simulink model "optimalswitching"  (R2024b)
settings: Solver=ode45  StartTime=0.0  StopTime=0.5  MaxStep=1e-7  MinStep=1e-8  RelTol=1e-6
values from neighbouring files (symbols this model uses):
  ma = 0.1    [three_level_parameter.m]
  Ts = 1/Fsw    (= 0.00111111111111)    [three_level_parameter.m]
  Vd = 400    [three_level_parameter.m]
  Vrefmax = Vdclink_max*cos(pi/6)    [three_level_parameter.m]
libraries: spsIGBTDiodeLib x12, spsDiodeLib x6, spsSeriesRLCLoadLib x3, spsDCVoltageSourceLib x2, spsGroundLib x1, spsThreePhaseVIMeasurementLib x1, sps_lib x1, simulink x1
settings SolverCC: ZeroCrossControl=DisableAll
settings DataIOCC: Refine=1000

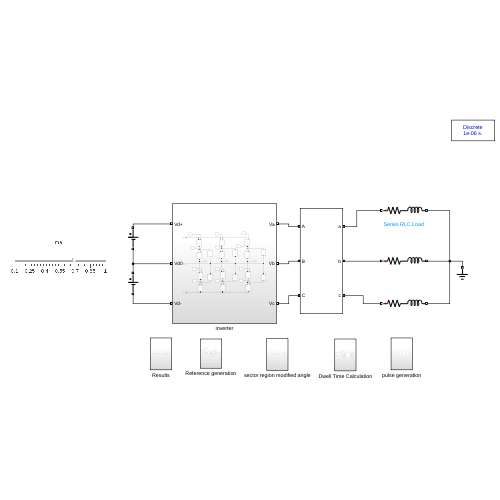
[thumbnail: Simulink's stored preview of the top-level diagram]
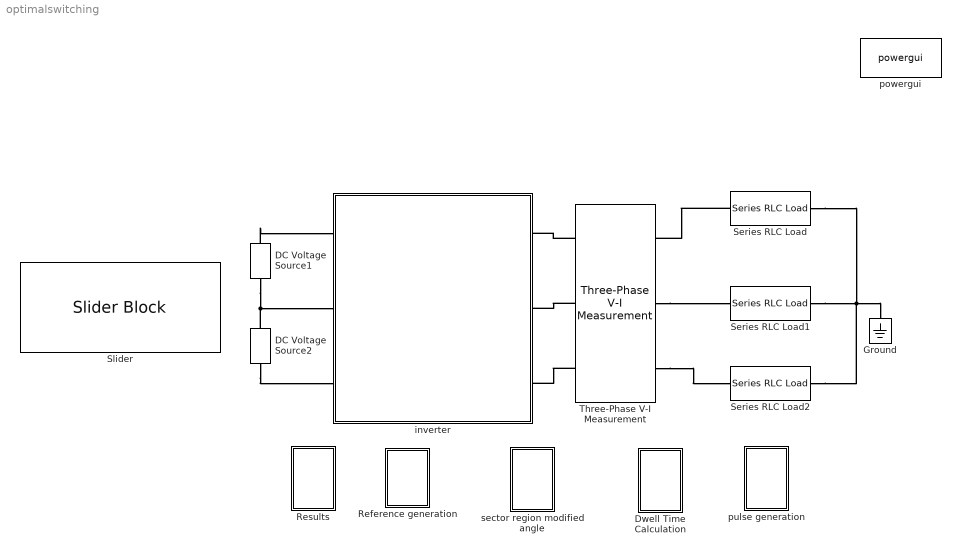
== system optimalswitching ==
  DC Voltage Source1 : spsDCVoltageSourceLib/DC Voltage Source  Amplitude=200  Measurements=None
  DC Voltage Source2 : spsDCVoltageSourceLib/DC Voltage Source  Amplitude=200  Measurements=None
  Dwell Time Calculation : Subsystem
  Ground : spsGroundLib/Ground  LConnTagsString=a
  Reference generation : Subsystem
  Results : Subsystem
  Series RLC Load : spsSeriesRLCLoadLib/Series RLC Load  LConnTagsString=a  RConnTagsString=__new0  NominalVoltage=240  NominalFrequency=50  ActivePower=1e3  InductivePower=484  CapacitivePower=0  Setx0=off  InitialVoltage=0  SetiL0=off  InitialCurrent=0  Measurements=None  LoadType=constant Z
  Series RLC Load1 : spsSeriesRLCLoadLib/Series RLC Load  LConnTagsString=a  RConnTagsString=__new0  NominalVoltage=240  NominalFrequency=50  ActivePower=1e3  InductivePower=484  CapacitivePower=0  Setx0=off  InitialVoltage=0  SetiL0=off  InitialCurrent=0  Measurements=None  LoadType=constant Z
  Series RLC Load2 : spsSeriesRLCLoadLib/Series RLC Load  LConnTagsString=a  RConnTagsString=__new0  NominalVoltage=240  NominalFrequency=50  ActivePower=1e3  InductivePower=484  CapacitivePower=0  Setx0=off  InitialVoltage=0  SetiL0=off  InitialCurrent=0  Measurements=None  LoadType=constant Z
  Slider : SliderBlock  ScaleMin=0.1  ScaleMax=1
  Three-Phase V-I Measurement : spsThreePhaseVIMeasurementLib/Three-Phase V-I Measurement  VoltageMeasurement=phase-to-ground  SetLabelV=on  LabelV=Vabc  Vpu=off  VpuLL=off  CurrentMeasurement=yes  SetLabelI=on  LabelI=Iabc  Ipu=off  Pbase=100e6  Vbase=500e3  OutputType=Complex  PhasorSimulation=off  PSBequivalent=0
  inverter : Subsystem
  powergui : sps_lib/powergui  Priority=1  SimulationMode=Discrete  SampleTime=1e-6  frequency=60  Iterations=50  frequencyindice=0  Pbase=100e6  ErrMax=1e-4  UnitsV=kV  UnitsW=MW  buscounter=0  FunctionMessages=off  echomessages=off  EnableUseOfTLC=off  CurrentSourceSwitches=off  DisableSnubberDevices=off  DisableRonSwitches=off  DisableVfSwitches=off  DisplayEquations=off  AutomaticDiscreteSolvers=off  SolverType=Tustin/Backward Euler (TBE)  Interpol=off  ExternalGateDelay=off  methode=off  Ts=100  x0status=blocks  SPID=on  SwTol=0  HookPort=off  NonlinearTolerance=1e-4  nMaxIteration=100  ContinueOnMaxIteration=off  RestoreLinks=warning  ResistiveCurrentMeasurement=off  Frange=[0:2:500]  Ylog=off  Xlog=on  ShowGrid=off  save=off  variable=ZData  structure=0  ZoomFFT=off  StartTime=0.0  cycles=1  DisplayStyle=1  fundamental=60  FreqAxis=off  MaxFrequency=1000  frequencyindicesteady=1  RmsSteady=1  display=off
  pulse generation : Subsystem
  sector region modified angle : Subsystem
  connections:
  Series RLC Load1/RConn1 -- Series RLC Load/RConn1 -- Ground/LConn1 -- Series RLC Load2/RConn1
  Three-Phase V-I Measurement/RConn3 -- Series RLC Load2/LConn1
  Series RLC Load/LConn1 -- Three-Phase V-I Measurement/RConn1
  Three-Phase V-I Measurement/RConn2 -- Series RLC Load1/LConn1
  Three-Phase V-I Measurement/LConn1 -- inverter/RConn1
  Three-Phase V-I Measurement/LConn2 -- inverter/RConn2
  Three-Phase V-I Measurement/LConn3 -- inverter/RConn3
  DC Voltage Source1/RConn1 -- inverter/LConn1
  DC Voltage Source1/LConn1 -- DC Voltage Source2/RConn1 -- inverter/LConn2
  DC Voltage Source2/LConn1 -- inverter/LConn3

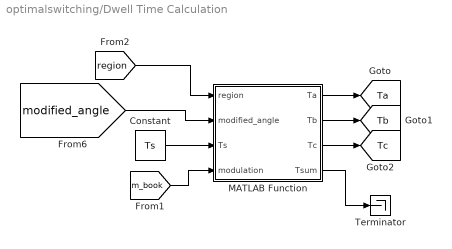
== system optimalswitching/Dwell Time Calculation ==
  Constant : Constant  Value=Ts
  MATLAB Function : MATLAB Function  TreatAsAtomicUnit=on
  Terminator : Terminator
  tag scope: Ta=global, Tb=global, Tc=global
  wires:
  [m_book] -> MATLAB Function/4(modulation)
  [region] -> MATLAB Function/1(region)
  Constant/1 -> MATLAB Function/3(Ts)
  [modified_angle] -> MATLAB Function/2(modified_angle)
  MATLAB Function/1(Ta) -> [Ta]
  MATLAB Function/2(Tb) -> [Tb]
  MATLAB Function/3(Tc) -> [Tc]
  MATLAB Function/4(Tsum) -> Terminator/1

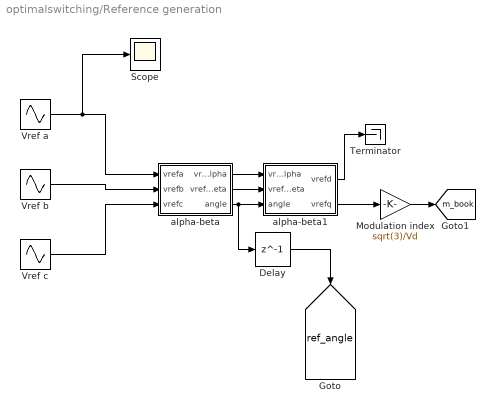
== system optimalswitching/Reference generation ==
  Delay : Delay  DelayLength=1  InitialCondition=0  SampleTime=Ts
  Modulation index : Gain  Gain=sqrt(3)/Vd
  Scope : Scope
  Terminator : Terminator
  Vref a : Sin  Amplitude=ma*Vrefmax  Frequency=2*pi*50  SampleTime=0
  Vref b : Sin  Amplitude=ma*Vrefmax  Frequency=2*pi*50  Phase=4*pi/3  SampleTime=0
  Vref c : Sin  Amplitude=ma*Vrefmax  Frequency=2*pi*50  Phase=2*pi/3  SampleTime=0
  alpha-beta : MATLAB Function  TreatAsAtomicUnit=on
  alpha-beta1 : MATLAB Function  TreatAsAtomicUnit=on
  tag scope: m_book=global, ref_angle=global
  wires:
  alpha-beta1/2(vrefq) -> Modulation index/1
  Vref b/1 -> alpha-beta/2(vrefb)
  alpha-beta/2(vrefbeta) -> alpha-beta1/2(vrefbeta)
  Vref c/1 -> alpha-beta/3(vrefc)
  Vref a/1 -> Scope/1, alpha-beta/1(vrefa)
  alpha-beta/3(angle) -> Delay/1, alpha-beta1/3(angle)
  Modulation index/1 -> [m_book]
  alpha-beta/1(vrefalpha) -> alpha-beta1/1(vrefalpha)
  alpha-beta1/1(vrefd) -> Terminator/1
  Delay/1 -> [ref_angle]

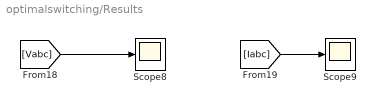
== system optimalswitching/Results ==
  Scope8 : Scope
  Scope9 : Scope
  wires:
  [Iabc] -> Scope9/1
  [Vabc] -> Scope8/1

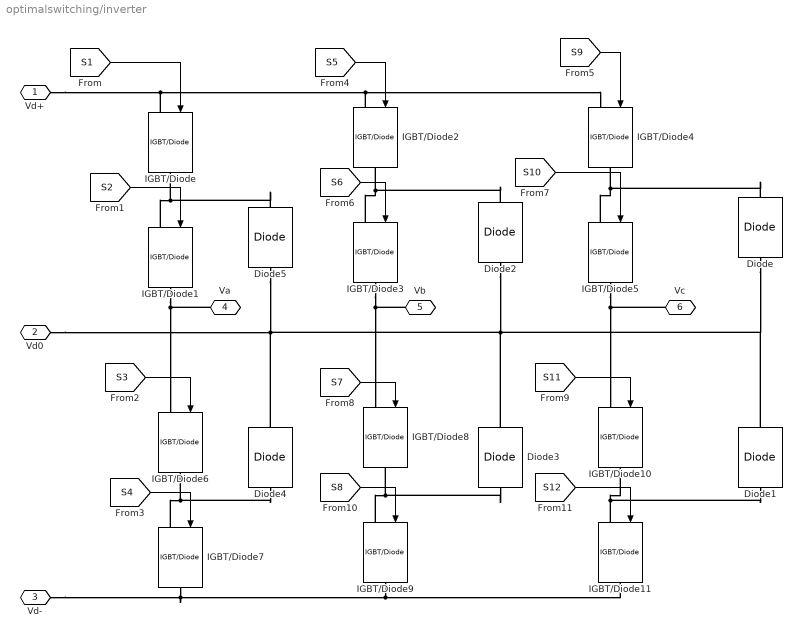
== system optimalswitching/inverter ==
  Diode{,1..5} (6 alike) : spsDiodeLib/Diode  Ron=0.001  Lon=0  Vf=0.8  IC=0  UseSnubber=0  Rs=500  Cs=250e-9  Measurements=off
  IGBT/Diode{,1..11} (12 alike) : spsIGBTDiodeLib/IGBT//Diode  Ron=1e-3  Rs=1e5  Cs=inf  Measurements=off
  Vd+ : PMIOPort  Side=Left
  Vd0 : PMIOPort  Port=2  Side=Left
  Vd- : PMIOPort  Port=3  Side=Left
  Va : PMIOPort  Port=4  Side=Right
  Vb : PMIOPort  Port=5  Side=Right
  Vc : PMIOPort  Port=6  Side=Right
  wires:
  [S1] -> IGBT/Diode/1
  [S3] -> IGBT/Diode6/1
  [S8] -> IGBT/Diode9/1
  [S7] -> IGBT/Diode8/1
  [S9] -> IGBT/Diode4/1
  [S12] -> IGBT/Diode11/1
  [S4] -> IGBT/Diode7/1
  [S10] -> IGBT/Diode5/1
  [S11] -> IGBT/Diode10/1
  [S5] -> IGBT/Diode2/1
  [S6] -> IGBT/Diode3/1
  [S2] -> IGBT/Diode1/1
  connections:
  Vd0/RConn1 -- Diode4/RConn1 -- Diode3/RConn1 -- Diode1/RConn1 -- Diode/LConn1 -- Diode2/LConn1 -- Diode5/LConn1
  IGBT/Diode3/RConn1 -- IGBT/Diode8/LConn1 -- Vb/RConn1
  IGBT/Diode5/RConn1 -- Vc/RConn1 -- IGBT/Diode10/LConn1
  IGBT/Diode11/LConn1 -- Diode1/LConn1 -- IGBT/Diode10/RConn1
  IGBT/Diode9/LConn1 -- Diode3/LConn1 -- IGBT/Diode8/RConn1
  IGBT/Diode1/RConn1 -- IGBT/Diode6/LConn1 -- Va/RConn1
  IGBT/Diode1/LConn1 -- Diode5/RConn1 -- IGBT/Diode/RConn1
  IGBT/Diode7/LConn1 -- Diode4/LConn1 -- IGBT/Diode6/RConn1
  IGBT/Diode/LConn1 -- Vd+/RConn1 -- IGBT/Diode2/LConn1 -- IGBT/Diode4/LConn1
  IGBT/Diode7/RConn1 -- Vd-/RConn1 -- IGBT/Diode9/RConn1 -- IGBT/Diode11/RConn1
  IGBT/Diode3/LConn1 -- Diode2/RConn1 -- IGBT/Diode2/RConn1
  IGBT/Diode5/LConn1 -- Diode/RConn1 -- IGBT/Diode4/RConn1

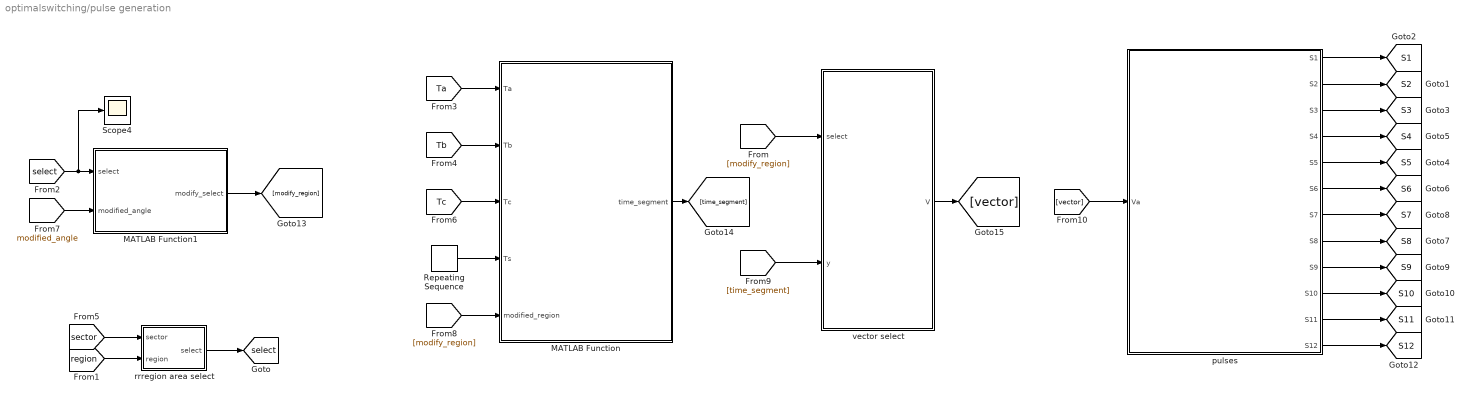
== system optimalswitching/pulse generation ==
  MATLAB Function : MATLAB Function  TreatAsAtomicUnit=on
  MATLAB Function1 : MATLAB Function  TreatAsAtomicUnit=on
  Repeating Sequence : simulink/Sources/Repeating Sequence  rep_seq_t=[0 Ts]  rep_seq_y=[0 Ts]
  Scope4 : Scope
  pulses : MATLAB Function  TreatAsAtomicUnit=on
  rrregion area select : MATLAB Function  TreatAsAtomicUnit=on
  vector select : MATLAB Function  TreatAsAtomicUnit=on
  tag scope: S10=global, S11=global, S12=global, S1=global, S2=global, S3=global, S4=global, S5=global, S6=global, S7=global, S8=global, S9=global, select=global
  wires:
  pulses/4(S4) -> [S4]
  [Tc] -> MATLAB Function/3(Tc)
  pulses/3(S3) -> [S3]
  pulses/1(S1) -> [S1]
  pulses/6(S6) -> [S6]
  [sector] -> rrregion area select/1(sector)
  pulses/5(S5) -> [S5]
  pulses/12(S12) -> [S12]
  pulses/7(S7) -> [S7]
  rrregion area select/1(select) -> [select]
  pulses/9(S9) -> [S9]
  [Ta] -> MATLAB Function/1(Ta)
  pulses/8(S8) -> [S8]
  [region] -> rrregion area select/2(region)
  Repeating Sequence/1 -> MATLAB Function/4(Ts)
  pulses/2(S2) -> [S2]
  pulses/10(S10) -> [S10]
  [Tb] -> MATLAB Function/2(Tb)
  pulses/11(S11) -> [S11]
  [select] -> Scope4/1, MATLAB Function1/1(select)
  [modified_angle] -> MATLAB Function1/2(modified_angle)
  MATLAB Function1/1(modify_select) -> [modify_region]
  [modify_region] -> vector select/1(select)
  [modify_region] -> MATLAB Function/5(modified_region)
  MATLAB Function/1(time_segment) -> [time_segment]
  [time_segment] -> vector select/2(y)
  vector select/1(V) -> [vector]
  [vector] -> pulses/1(Va)

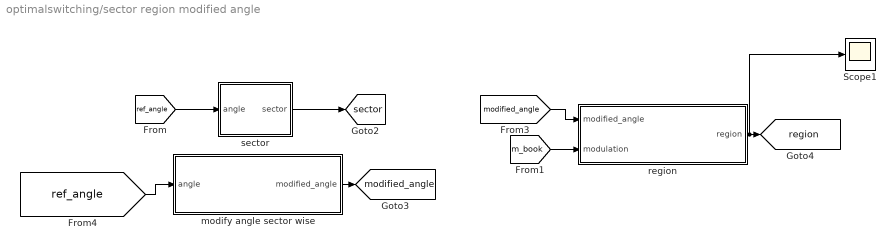
== system optimalswitching/sector region modified angle ==
  Scope1 : Scope
  modify angle sector wise : MATLAB Function  TreatAsAtomicUnit=on
  region : MATLAB Function  TreatAsAtomicUnit=on
  sector : MATLAB Function  TreatAsAtomicUnit=on
  tag scope: modified_angle=global, region=global, sector=global
  wires:
  [ref_angle] -> modify angle sector wise/1(angle)
  modify angle sector wise/1(modified_angle) -> [modified_angle]
  region/1(region) -> Scope1/1, [region]
  sector/1(sector) -> [sector]
  [m_book] -> region/2(modulation)
  [ref_angle] -> sector/1(angle)
  [modified_angle] -> region/1(modified_angle)

== matlab function optimalswitching/pulse generation/MATLAB Function ==
  data: Ta input; time_segment output; Tb input; Tc input; Ts input; modified_region input
function time_segment = fcn(Ta,Tb,Tc,Ts,modified_region)
a= Ta*0.25;
b= a+Tb*0.5;
c= b+Tc*0.5;
d= c+Ta*0.5;
e= d+Tc*0.5;
f= e+Tb*0.5;
g= f+Ta*0.25;

aa= Tc*0.25;
bb= aa+Tb*0.5;
cc= bb+Ta*0.5;
dd= cc+Tc*0.5;
ee= dd+Ta*0.5;
ff= ee+Tb*0.5;
gg= ff+Tc*0.25;
if(modified_region==111 || modified_region==121|| modified_region==211 || modified_region ==221 ||modified_region==311 ||modified_region==321 ||modified_region==411 || modified_region==421 ||modified_region==511||modified_region==521 || modified_region ==611||modified_region==621||modified_region==13||modified_region==23||modified_region==33||modified_region==43||modified_region==53||modified_region==63)
    if(a>=Ts)
        time_segment=1;
    elseif(b>=Ts && Ts>a)
        time_segment=2;
    elseif(c>=Ts && Ts>b)
        time_segment=3;
    elseif(d>=Ts && Ts>c)
        time_segment=4;
    elseif(e>=Ts && Ts>d)
        time_segment=5;
    elseif(f>=Ts && Ts>e)
        time_segment=6;
    elseif(g>=Ts && Ts>f)
        time_segment=7;
    else
        time_segment=0;
    end
else
    if(aa>=Ts)
        time_segment=8;
    elseif(bb>=Ts && Ts>aa)
        time_segment=9;
    elseif(cc>=Ts && Ts>bb)
        time_segment=10;
    elseif(dd>=Ts && Ts>cc)
        time_segment=11;
    elseif(ee>=Ts && Ts>dd)
        time_segment=12;
    elseif(ff>=Ts && Ts>ee)
        time_segment=13;
    elseif(gg>=Ts && Ts>ff)
        time_segment=14;
    else
        time_segment=0;
    end
end

== matlab function optimalswitching/pulse generation/MATLAB Function1 ==
  data: select input; modify_select output; modified_angle input
function modify_select = fcn(select,modified_angle)

if(select==11 && modified_angle<pi/6)
    modify_select= 111; %Sector 1 Region 1 and Subsector a
elseif(select==11 && modified_angle>pi/6 && modified_angle<=pi/3)
    modify_select= 112; %Sector 1 Region 1 and Subsector b
elseif(select==12 && modified_angle<pi/6)
    modify_select= 121; %Sector 1 Region 2 and Subsector a
elseif(select==12 && modified_angle>pi/6 && modified_angle<=pi/3)
    modify_select= 122; %Sector 1 Region 2 and Subsector b
elseif(select==21 && modified_angle<pi/6)
    modify_select= 211; %Sector 2 Region 1 and Subsector a
elseif(select==21 && modified_angle>pi/6 && modified_angle<=pi/3)
    modify_select= 212; %Sector 2 Region 1 and Subsector b
elseif(select==22 && modified_angle<pi/6)
    modify_select= 221; %Sector 2 Region 2 and Subsector a
elseif(select==22 && modified_angle>pi/6 && modified_angle<=pi/3)
    modify_select= 222; %Sector 2 Region 2 and Subsector b
elseif(select==31 && modified_angle<pi/6)
    modify_select= 311; %Sector 3 Region 1 and Subsector a
elseif(select==31 && modified_angle>pi/6 && modified_angle<=pi/3)
    modify_select= 312; %Sector 3 Region 1 and Subsector b
elseif(select==32 && modified_angle<pi/6)
    modify_select= 321; %Sector 3 Region 2 and Subsector a
elseif(select==32 && modified_angle>pi/6 && modified_angle<=pi/3)
    modify_select= 322; %Sector 3 Region 2 and Subsector b
elseif(select==41 && modified_angle<pi/6)
    modify_select= 411; %Sector 4 Region 1 and Subsector a
elseif(select==41 && modified_angle>pi/6 && modified_angle<=pi/3)
    modify_select= 412; %Sector 4 Region 1 and Subsector b
elseif(select==42 && modified_angle<pi/6)
    modify_select= 421; %Sector 4 Region 2 and Subsector a
elseif(select==42 && modified_angle>pi/6 && modified_angle<=pi/3)
    modify_select= 422; %Sector 4 Region 2 and Subsector b
elseif(select==51 && modified_angle<pi/6)
    modify_select= 511; %Sector 5 Region 1 and Subsector a
elseif(select==51 && modified_angle>pi/6 && modified_angle<=pi/3)
    modify_select= 512; %Sector 5 Region 1 and Subsector b
elseif(select==52 && modified_angle<pi/6)
    modify_select= 521; %Sector 5 Region 2 and Subsector a
elseif(select==52 && modified_angle>pi/6 && modified_angle<=pi/3)
    modify_select= 522; %Sector 5 Region 2 and Subsector b
elseif(select==61 && modified_angle<pi/6)
    modify_select= 611; %Sector 6 Region 1 and Subsector a
elseif(select==61 && modified_angle>pi/6 && modified_angle<=pi/3)
    modify_select= 612; %Sector 6 Region 1 and Subsector b
elseif(select==62 && modified_angle<pi/6)
    modify_select= 621; %Sector 6 Region 2 and Subsector a
elseif(select==62 && modified_angle>pi/6 && modified_angle<=pi/3)
    modify_select= 622; %Sector 6 Region 2 and Subsector b
else
    modify_select=select;
end

== matlab function optimalswitching/Reference generation/alpha-beta1 ==
  data: vrefalpha input; vrefd output; vrefbeta input; angle input; vrefq output
function [vrefd,vrefq] = fcn(vrefalpha,vrefbeta,angle)

vrefd = vrefalpha*cos(angle)-vrefbeta*sin(angle);
vrefq= vrefalpha*sin(angle)+vrefbeta*cos(angle);

== matlab function optimalswitching/Reference generation/alpha-beta ==
  data: vrefa input; vrefalpha output; vrefb input; vrefc input; vrefbeta output; angle output
function [vrefalpha,vrefbeta,angle] = fcn(vrefa,vrefb,vrefc)

vrefalpha= 2*(vrefa-0.5*vrefb-0.5*vrefc)/3;
vrefbeta= (-vrefb+vrefc)*sqrt(3)/3;
ang= atan2(vrefalpha,vrefbeta);
if(ang>=0 && ang<=pi)
    angle=ang;
else
    angle=2*pi+ang;
end

== matlab function optimalswitching/sector region modified angle/sector ==
  data: sector output; angle input
function sector  = fcn(angle)

if(angle>=0 && angle<pi/3)
    sector=1;
elseif (angle>=pi/3 && angle< 2*pi/3)
    sector=2;
elseif (angle>=2*pi/3 && angle< 3*pi/3)
    sector=3;
elseif (angle>=3*pi/3 && angle< 4*pi/3)
    sector=4;
elseif (angle>=4*pi/3 && angle< 5*pi/3)
    sector=5;
elseif (angle>=5*pi/3 && angle<= 2*pi)
    sector=6;
else
    sector=1;
end

== matlab function optimalswitching/sector region modified angle/modify angle sector wise ==
  data: modified_angle output; angle input
function modified_angle  = fcn(angle)

if(angle>=0 && angle<pi/3)
    modified_angle=angle;
elseif (angle>=pi/3 && angle< 2*pi/3)
    modified_angle=angle-pi/3;
elseif (angle>=2*pi/3 && angle< 3*pi/3)
    modified_angle=angle-2*pi/3;
elseif (angle>=3*pi/3 && angle< 4*pi/3)
    modified_angle=angle-3*pi/3;
elseif (angle>=4*pi/3 && angle< 5*pi/3)
    modified_angle=angle-4*pi/3;
else
    modified_angle=angle-5*pi/3;
end

== matlab function optimalswitching/sector region modified angle/region ==
  data: region output; modified_angle input; modulation input
function region  = fcn(modified_angle, modulation)
m1= modulation*(sqrt(3)*cos(modified_angle)-sin(modified_angle))/2;
m2= modulation*sin(modified_angle);

if(m1>=0.5)
    region=3;
elseif(m2>=0.5)
    region=4;
elseif(m1+m2<=0.5 && m1<0.5 && m2<0.5)
    region=1;
else
    region=2;
end

== matlab function optimalswitching/Dwell Time Calculation/MATLAB Function ==
  data: region input; Ta output; modified_angle input; Ts input; Tb output; Tc output; modulation input; Tsum output
function [Ta,Tb,Tc,Tsum] = fcn(region,modified_angle,Ts,modulation)
if(region==1)
    Ta = Ts*(2*modulation*sin((pi/3)-modified_angle));
    Tb= Ts*(1-2*modulation*sin((pi/3)+modified_angle));
    Tc=Ts*(2*modulation*sin(modified_angle)); 
elseif(region==2)
    Ta = Ts*(1-2*modulation*sin(modified_angle));
    Tb= -Ts*(1-2*modulation*sin((pi/3)+modified_angle));
    Tc=Ts*(1-2*modulation*sin((pi/3)-modified_angle)); 
elseif(region==3)
    Ta = Ts*(2-2*modulation*sin((pi/3)+modified_angle));
    Tb= Ts*(2*modulation*sin(modified_angle));
    Tc=-Ts*(1-2*modulation*sin((pi/3)-modified_angle));
elseif(region==4)
    Ta= Ts*(2*modulation*sin(modified_angle)-1);
    Tb = Ts*(2*modulation*sin((pi/3)-modified_angle));
    Tc = Ts*(2-2*modulation*sin((pi/3)+modified_angle));
else
    Ta=0;
    Tb=0;
    Tc=0;
end
Tsum=Ta+Tb+Tc;

== matlab function optimalswitching/pulse generation/rrregion area select ==
  data: sector input; region input; select output
function select= fcn(sector,region)
% select variable 1st number denotes sector 2nd number denotes region
if(sector==1)
    if(region==1)
        select=11;
    elseif(region==2)
        select=12;
    elseif(region==3)
        select=13;
    else
        select=14;
    end
elseif(sector==2)
    if(region==1)
        select=21;
    elseif(region==2)
        select=22;
    elseif(region==3)
        select=23;
    else
        select=24;
    end
elseif(sector==3)
    if(region==1)
        select=31;
    elseif(region==2)
        select=32;
    elseif(region==3)
        select=33;
    else
        select=34;
    end
elseif(sector==4)
    if(region==1)
        select=41;
    elseif(region==2)
        select=42;
    elseif(region==3)
        select=43;
    else
        select=44;
    end
elseif(sector==5)
    if(region==1)
        select=51;
    elseif(region==2)
        select=52;
    elseif(region==3)
        select=53;
    else
        select=54;
    end
else
    if(region==1)
        select=61;
    elseif(region==2)
        select=62;
    elseif(region==3)
        select=63;
    else
        select=64;
    end
end

== matlab function optimalswitching/pulse generation/vector select ==
  data: select input; V output; y input
function V = fcn(select,y)
V0a= [3,3,3]; %PPP
V0b= [2,2,2]; %OOO
V0c= [1,1,1]; %NNN
V1a= [3,2,2]; %POO
V1b= [2,1,1]; %ONN
V2a= [3,3,2]; %PPO
V2b= [2,2,1];%OON
V3a= [2,3,2];%OPO
V3b= [1,2,1];%NON
V4a= [2,3,3];%OPP
V4b= [1,2,2];%NOO
V5a= [2,2,3];%OOP 
V5b= [1,1,2];%NNO
V6a= [3,2,3];%POP
V6b= [2,1,2];%ONO
V7= [3,2,1]; %PON
V8= [2,3,1]; %OPN
V9= [1,3,2];%NPO
V10= [1,2,3];%NOP
V11= [2,1,3];%ONP
V12= [3,1,2];%PNO
V13= [3,1,1];%PNN
V14= [3,3,1];%PPN
V15= [1,3,1];%NPN
V16= [1,3,3];%NPP
V17= [1,1,3];%NNP
V18= [3,1,3];%PNP
%%%%%%%%%%%%%%%%% Sector 1 %%%%%%%%%%%%%%%%%%%%%%%
if(select==111)
    Va=V1a;
    Vb=V0b;
    Vc=V2b;
    Vd=V1b;
elseif(select==112)
    Va=V1a;
    Vb=V0b;
    Vc=V2b;
    Vd=V2a;

elseif(select==121)
    Va= V1a;
    Vb= V7;
    Vc=V2b;
    Vd=V1b;
elseif(select==122)
    Va= V1a;
    Vb= V7;
    Vc=V2b;
    Vd=V2a;

elseif(select==13)
    Va= V1a;
    Vb= V7;
    Vc=V13;
    Vd=V1b;

elseif(select==14)
    Va= V14;
    Vb= V7;
    Vc=V2b;
    Vd=V2a;
%%%%%%%%%%%%%%%%%% Sector 2 %%%%%%%%%%%%%%%%%%
elseif(select==211)
    Va= V2b;
    Vb= V0b;
    Vc= V3a; 
    Vd= V2a;
elseif(select==212)
    Va= V2b;
    Vb= V0b;
    Vc= V3a; 
    Vd= V3b;
elseif(select==221)
    Va= V2b;
    Vb= V8;
    Vc= V3a; 
    Vd= V2a;
elseif(select==222)
    Va= V2b;
    Vb= V8;
    Vc= V3a; 
    Vd= V3b;
elseif(select==23)
    Va= V2b;
    Vb= V8;
    Vc=V14;
    Vd= V2a;
elseif(select==24)
    Va= V15;
    Vb= V8;
    Vc=V3a;
    Vd=V3b;
%%%%%%%%%%%%%%%%%%%% Sector 3 %%%%%%%%%%%%%%%%%%%%%%
elseif(select==311)
    Va= V3a;
    Vb= V0b;
    Vc=V4b;
    Vd=V3b;
elseif(select==312)
    Va= V3a;
    Vb= V0b;
    Vc=V4b;
    Vd=V4a;
elseif(select==321)
    Va= V3a;
    Vb= V9;
    Vc=V4b;
    Vd= V3b;

elseif(select==322)
    Va= V3a;
    Vb= V9;
    Vc=V4b;
    Vd= V4a;

elseif(select==33)
    Va= V3a;
    Vb= V9;
    Vc=V15;
    Vd=V3b;

elseif(select==34)
    Va= V16;
    Vb= V9;
    Vc=V4b;
    Vd=V4a;
 %%%%%%%%%%%%%%%%%%%%% Sector 4 %%%%%%%%%%%%%%%%%%%%%
elseif(select==411)
    Va= V4b;
    Vb= V0b;
    Vc=V5a; 
    Vd= V4a;
elseif(select==412)
    Va= V4b;
    Vb= V0b;
    Vc=V5a; 
    Vd= V5b;

elseif(select==421)
    Va= V4b;
    Vb= V10;
    Vc=V5a; 
    Vd= V4a;
elseif(select==422)
    Va= V4b;
    Vb= V10;
    Vc=V5a; 
    Vd= V5b;
elseif(select==43)
    Va= V4b;
    Vb= V10;
    Vc=V16; 
    Vd= V4a;

elseif(select==44)
    Va= V17;
    Vb= V10;
    Vc=V5a; 
    Vd=V5b;

%%%%%%%%%%%%%%%%%%%% Sector 5 %%%%%%%%%%%%%%%%%%%%%%%%%

elseif(select==511)
    Va= V5a;
    Vb= V0b;
    Vc=V6b; 
    Vd= V5b;
elseif(select==512)
    Va= V5a;
    Vb= V0b;
    Vc=V6b; 
    Vd= V6a;

elseif(select==521)
    Va= V5a;
    Vb= V11;
    Vc=V6b; 
    Vd= V5b;
elseif(select==522)
    Va= V5a;
    Vb= V11;
    Vc=V6b; 
    Vd= V6a;
elseif(select==53)
    Va= V5a;
    Vb= V11;
    Vc=V17; 
    Vd= V5b;

elseif(select==54)
    Va= V18;
    Vb= V11;
    Vc=V6b; 
    Vd=V6a;
%%%%%%%%%%%%%%%%%%%%%%%% Sector 6 %%%%%%%%%%%%%%%%%%%%%%%%%%%
elseif(select==611)
    Va= V6b;
    Vb= V0b;
    Vc=V1a; 
    Vd= V6a;
elseif(select==612)
    Va= V6b;
    Vb= V0b;
    Vc=V1a; 
    Vd= V1b;

elseif(select==621)
    Va= V6b;
    Vb= V12;
    Vc=V1a; 
    Vd= V6a;
elseif(select==622)
    Va= V6b;
    Vb= V12;
    Vc=V1a; 
    Vd= V1b;
elseif(select==63)
    Va= V6b;
    Vb= V12;
    Vc=V18; 
    Vd= V6a;

elseif(select==64)
    Va= V13;
    Vb= V12;
    Vc=V1a; 
    Vd=V1b;
else
    Va=V0a;
    Vb=V0b;
    Vc=V0c;
    Vd=V0a;
end

if(y==1)
    V=Va;
elseif(y==2)
    V=Vb;
elseif(y==3)
    V=Vc;
elseif(y==4)
    V=Vd;
elseif(y==5)
    V=Vc;
elseif(y==6)
    V=Vb;
elseif(y==7)
    V=Va;
elseif(y==8)
    V=Vc;
elseif(y==9)
    V=Vb;
elseif(y==10)
    V=Va;
elseif(y==11)
    V=Vd;
elseif(y==12)
    V=Va;
elseif (y==13)
    V=Vb;
elseif(y==14)
    V=Vc;
else
    V=V0a;
end

== matlab function optimalswitching/pulse generation/pulses ==
  data: Va input; S1 output; S2 output; S3 output; S4 output; S5 output; S6 output; S7 output; S8 output; S9 output; S10 output; S11 output; S12 output
function [S1,S2,S3,S4,S5,S6,S7,S8,S9,S10,S11,S12]= fcn(Va)


if(Va(1)==3)
    S1=1;
    S2=1;
    S3=0;
    S4=0;
elseif(Va(1)==2)
    S1=0;
    S2=1;
    S3=1;
    S4=0;
else
    S1=0;
    S2=0;
    S3=1;
    S4=1;
end
if(Va(2)==3)
    S5=1;
    S6=1;
    S7=0;
    S8=0;
elseif(Va(2)==2)
    S5=0;
    S6=1;
    S7=1;
    S8=0;
else
    S5=0;
    S6=0;
    S7=1;
    S8=1;
end
if(Va(3)==3)
    S9=1;
    S10=1;
    S11=0;
    S12=0;
elseif(Va(3)==2)
    S9=0;
    S10=1;
    S11=1;
    S12=0;
else
    S9=0;
    S10=0;
    S11=1;
    S12=1;
end
